simulink model "pahrah"  (Simulink 3.00)
settings: Solver=ode15s  SolverMode=SingleTasking  StartTime=0.0  StopTime=60  MaxStep=5  RelTol=1e-6  AbsTol=1e-6
undefined symbols (not defined in the file): Aail, Aelv, Arud, Bail, Belv, Brud, Cail, Celv, Crud, Dail, dar, Delv, drr, Drud, Ki_1, Ki_2, Kphi, Kq, Kr, Ktheta, uaero0, uprop0, xinco
libraries: fbuttons x1, fdclib10 x1
settings Model: SaveTime=off  SaveOutput=off  RTWTemplateMakefile=grt_vc.tmf  LastModifiedBy=Dutchroll

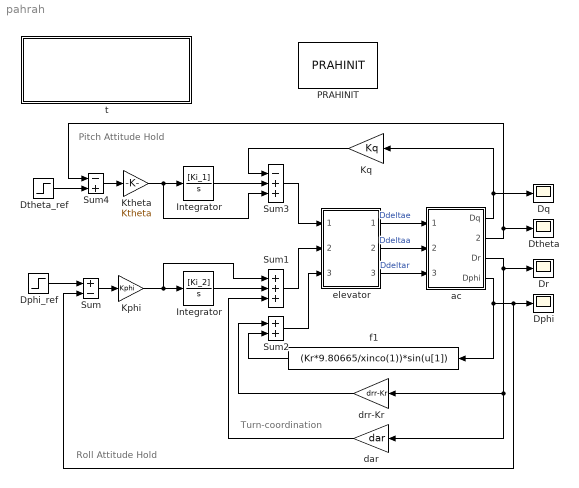
== system pahrah ==
  note: Roll Attitude Hold
  note: Pitch Attitude Hold
  note: Turn-coordination
  Dphi : Scope
      settings: TickLabels=on  TimeRange=60.000000  YMin=-0.3  YMax=0.3  SaveToWorkspace=off  SaveName=ScopeData  DataFormat=Matrix
  Dphi_ref : Step  Time=0  Before=0  After=10*pi/180  SampleTime=0
  Dq : Scope
      settings: TickLabels=on  TimeRange=60.000000  YMin=-0.03  YMax=0.03  SaveToWorkspace=off  SaveName=ScopeData  DataFormat=Matrix
  Dr : Scope
      settings: TickLabels=on  TimeRange=60.000000  YMin=-0.025  YMax=0.025  SaveToWorkspace=off  SaveName=ScopeData  DataFormat=Matrix
  Dtheta : Scope
      settings: TickLabels=on  TimeRange=60.000000  YMin=-0.025  YMax=0.025  SaveToWorkspace=off  SaveName=ScopeData  DataFormat=Matrix
  Dtheta_ref : Step  Time=0  Before=0  After=1*pi/180  SampleTime=0
  Integrator : TransferFcn  Numerator=[Ki_2]  Denominator=[1 0]
  "Integrator " : TransferFcn  Numerator=[Ki_1]  Denominator=[1 0]
  Kphi : Gain  Gain=Kphi  SaturateOnIntegerOverflow=on
  Kq : Gain  Orientation=left  Gain=Kq  SaturateOnIntegerOverflow=on
  Ktheta : Gain  Gain=Ktheta  SaturateOnIntegerOverflow=on
  PRAHINIT : fbuttons/PRAHINIT
  Sum : Sum  Inputs=+-  SaturateOnIntegerOverflow=on
  Sum1 : Sum  Inputs=+++  SaturateOnIntegerOverflow=on
  Sum2 : Sum  Inputs=++  SaturateOnIntegerOverflow=on
  Sum3 : Sum  Inputs=-++  SaturateOnIntegerOverflow=on
  Sum4 : Sum  Inputs=-+  SaturateOnIntegerOverflow=on
  ac : Subsystem
      mask Display: disp('BEAVER\ndynamics')
  dar : Gain  Orientation=left  Gain=dar  SaturateOnIntegerOverflow=on
  drr-Kr : Gain  Orientation=left  Gain=drr-Kr  SaturateOnIntegerOverflow=on
  elevator : Subsystem
      mask Display: disp('Cable &\nactuator\ndynamics')
  f1 : Fcn  Orientation=left  Expr=(Kr*9.80665/xinco(1))*sin(u[1])
  t : Subsystem
      settings: OpenFcn=browse apilot
      mask Display: disp('PAH without turn-compensation;\nRAH with turn-coordination\n(no signal limiters).\nMarc Rauw, May 2004')
  wires:
  ac/1(Dq) -> Dq/1, Kq/1
  ac/2(Dtheta) -> Dtheta/1, Sum4/1
  ac/3(Dr) -> Dr/1, dar/1, drr-Kr/1
  ac/4(Dphi) -> Sum/2, Dphi/1, f1/1
  elevator/3(Ddeltar) -> ac/3(Ddelta_r)  "Ddeltar"
  elevator/2(Ddeltaa) -> ac/2(Ddelta_a)  "Ddeltaa"
  elevator/1(Ddeltae) -> ac/1(Ddelta_e)  "Ddeltae"
  Dphi_ref/1 -> Sum/1
  Sum/1 -> Kphi/1
  drr-Kr/1 -> Sum2/1
  Sum2/1 -> elevator/3(VDdeltar)
  dar/1 -> Sum1/3
  Sum4/1 -> Ktheta/1
  Dtheta_ref/1 -> Sum4/2
  Sum3/1 -> elevator/1(VDdeltae)
  Kq/1 -> Sum3/1
  Sum1/1 -> elevator/2(VDdeltaa)
  "Integrator "/1 -> Sum3/2
  Ktheta/1 -> "Integrator "/1, Sum3/3
  Integrator/1 -> Sum1/2
  Kphi/1 -> Integrator/1, Sum1/1
  f1/1 -> Sum2/2

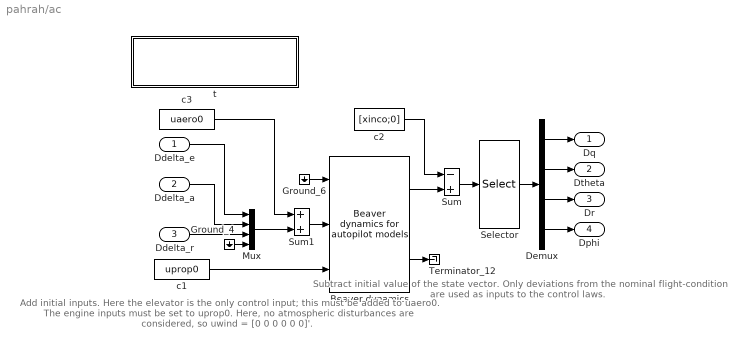
== system pahrah/ac ==
  note: Add initial inputs. Here the elevator
      | is the only control input; this must
      | be added to uaero0. The engine
      | inputs must be set to uprop0. Here,
      | no atmospheric disturbances are
      | considered, so uwind = [0 0 0 0 0 0]'.
  note: Subtract initial value of  the state
      | vector. Only deviations from the
      | nominal flight-condition are used
      | as inputs to the control laws.
  Ddelta_e : Inport  Port=1  PortWidth=-1  SampleTime=-1  DataType=auto
      settings: SignalType=auto
  Ddelta_a : Inport  Port=2  PortWidth=-1  SampleTime=-1  DataType=auto
      settings: SignalType=auto
  Ddelta_r : Inport  Port=3  PortWidth=-1  SampleTime=-1  DataType=auto
      settings: SignalType=auto
  Beaver dynamics : fdclib10/Beaver dynamics for autopilot models
  Demux : Demux  Outputs=4
  Ground_4 : Ground
  Ground_6 : Ground
  Mux : Mux  Inputs=4
      settings: DisplayOption=none
  Selector : Selector  Elements=[5 8 6 9]  InputPortWidth=13
  Sum : Sum  Inputs=-+  SaturateOnIntegerOverflow=on
  Sum1 : Sum  Inputs=++  SaturateOnIntegerOverflow=on
  Terminator_12 : Terminator
  c1 : Constant  Value=uprop0
  c2 : Constant  Value=[xinco;0]
  c3 : Constant  Value=uaero0
  t : Subsystem
      mask Display: disp('Call aircraft model and convert\nI/O signals to small-deviations.\nM.O. Rauw, January 2004')
  Dq : Outport  Port=1
  Dtheta : Outport  Port=2
  Dr : Outport  Port=3
  Dphi : Outport  Port=4
  wires:
  Beaver dynamics/1 -> Sum/2
  c2/1 -> Sum/1
  Beaver dynamics/2 -> Terminator_12/1
  Ddelta_e/1 -> Mux/1
  Ground_4/1 -> Mux/4
  Ddelta_r/1 -> Mux/3
  Ddelta_a/1 -> Mux/2
  Mux/1 -> Sum1/2
  c3/1 -> Sum1/1
  Sum1/1 -> Beaver dynamics/2
  c1/1 -> Beaver dynamics/3
  Sum/1 -> Selector/1
  Ground_6/1 -> Beaver dynamics/1
  Selector/1 -> Demux/1
  Demux/1 -> Dq/1
  Demux/2 -> Dtheta/1
  Demux/3 -> Dr/1
  Demux/4 -> Dphi/1

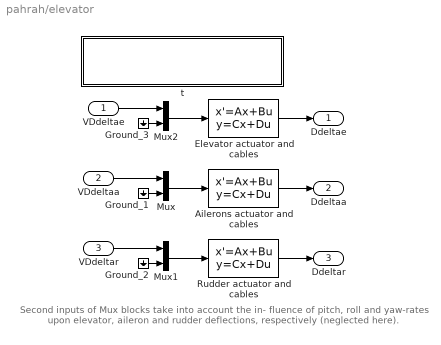
== system pahrah/elevator ==
  note: Second inputs of Mux blocks take into account the in-
      | fluence of pitch, roll and yaw-rates upon elevator, aileron
      | and rudder deflections, respectively (neglected here).
  VDdeltae : Inport  Port=1  PortWidth=-1  SampleTime=-1  DataType=auto
      settings: SignalType=auto
  VDdeltaa : Inport  Port=2  PortWidth=-1  SampleTime=-1  DataType=auto
      settings: SignalType=auto
  VDdeltar : Inport  Port=3  PortWidth=-1  SampleTime=-1  DataType=auto
      settings: SignalType=auto
  Ailerons actuator and cables : StateSpace  A=Aail  B=Bail  C=Cail  D=Dail  X0=0
  Elevator actuator and cables : StateSpace  A=Aelv  B=Belv  C=Celv  D=Delv  X0=0
  Ground_1 : Ground
  Ground_2 : Ground
  Ground_3 : Ground
  Mux : Mux  Inputs=2
      settings: DisplayOption=none
  Mux1 : Mux  Inputs=2
      settings: DisplayOption=none
  Mux2 : Mux  Inputs=2
      settings: DisplayOption=none
  Rudder actuator and cables : StateSpace  A=Arud  B=Brud  C=Crud  D=Drud  X0=0
  t : Subsystem
      settings: OpenFcn=browse actuatr
      mask Display: disp('Dynamics of the actuators and cables\nfor elevator, ailerons, and rudder.\nM.O. Rauw, April 2003')
  Ddeltae : Outport  Port=1
  Ddeltaa : Outport  Port=2
  Ddeltar : Outport  Port=3
  wires:
  Ailerons actuator and cables/1 -> Ddeltaa/1
  VDdeltaa/1 -> Mux/1
  Mux/1 -> Ailerons actuator and cables/1
  Mux1/1 -> Rudder actuator and cables/1
  VDdeltar/1 -> Mux1/1
  Rudder actuator and cables/1 -> Ddeltar/1
  Ground_1/1 -> Mux/2
  Ground_2/1 -> Mux1/2
  Elevator actuator and cables/1 -> Ddeltae/1
  Ground_3/1 -> Mux2/2
  Mux2/1 -> Elevator actuator and cables/1
  VDdeltae/1 -> Mux2/1

== system pahrah/t ==

== system pahrah/ac/t ==

== system pahrah/elevator/t ==
